simulink model "strain_gauge"  (R2019b)
settings: Solver=ode15s  StartTime=0.0  StopTime=100  RelTol=1e-3  AbsTol=1e-3  EnableMultiTasking=on
libraries: fl_lib x13, ee_lib x6, nesl_utility x3, simulink x1, dspsigops x1
Description:
  | Strain Gauge and Wheatstone Bridge
settings Model: ExtModeAutoUpdateStatusClock=off  Creator=The MathWorks, Inc.  LastModifiedBy=upattacini
settings SolverCC: AutoScaleAbsTol=off
settings DataIOCC: MaxDataPoints=10000  SaveOutput=off  SignalLogging=off  DSMLogging=off  SaveTime=off  ReturnWorkspaceOutputs=off  SignalLoggingName=logsout_ee_strain_gauge  Refine=5
settings OptimizationCC: ExpressionDepthLimit=2147483647  InitFltsAndDblsToZero=on  LifeSpan=inf
settings DebuggingCC: SaveWithParameterizedLinksMsg=none  UnderspecifiedInitializationDetection=Classic  MergeDetectMultiDrivingBlocksExec=none  SignalResolutionControl=TryResolveAllWithWarning  FcnCallInpInsideContextMsg=warning  StateNameClashWarn=warning  SFUnexpectedBacktrackingDiag=warning  SFNoUnconditionalDefaultTransitionDiag=warning  SFExecutionAtInitializationDiag=none  ArithmeticOperatorsInVariantConditions=warning
settings HardwareCC: ProdBitPerPointer=32  ProdBitPerSizeT=32  ProdBitPerPtrDiffT=32  ProdLargestAtomicFloat=None  ProdIntDivRoundTo=Undefined  ProdEndianess=Unspecified  ProdWordSize=32  ProdHWDeviceType=32-bit Generic
settings ModelReferenceCC: PropagateSignalLabelsOutOfModel=off
settings SFSimCC: SimUseLocalCustomCode=off  CustomCodeUndefinedFunction=UseInterfaceOnly
settings RTWCC: RTWUseLocalCustomCode=off
settings CodeAppCC: StateflowObjectComments=on
settings GRTTargetCC: TargetFcnLib=ansi_tfl_tmw.mat  TargetLangStandard=C89/C90 (ANSI)  GeneratePreprocessorConditionals=Disable all  CombineOutputUpdateFcns=off  GRTInterface=on
settings ConfigComp: CovMetricSettings=dw  CovHtmlReporting=on  CovSaveCumulativeToWorkspaceVar=on  CovSaveSingleToWorkspaceVar=on  CovExternalEMLEnable=off  CovSFcnEnable=off
settings SimscapeCC: SimscapeLogName=simlog_ee_strain_gauge  SimscapeLogDataHistory=10000

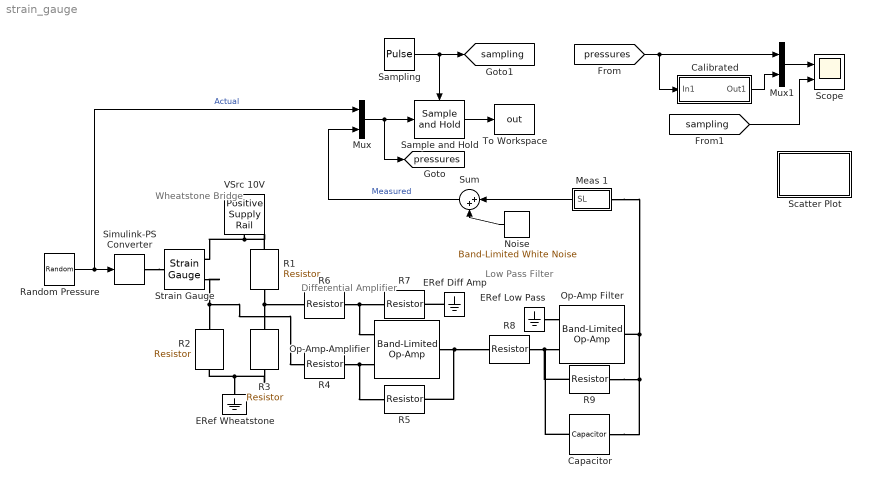
== system strain_gauge ==
  note: Low Pass Filter
  note: Differential Amplifier
  note: Wheatstone
      | Bridge
  Calibrated : Subsystem  mask{Switch=off, Gain=0.838, Bias=-8.5e-6}
      mask prompts: Switch "Enable Calibration"
      mask Callback Switch:
      | sw = get_param(gcb,'Switch');
      | if strcmp(sw,'on')
      |     set_param(gcb,'MaskEnableString','on,on,on');
      | else
      |     set_param(gcb,'MaskEnableString','on,off,off');
      | end
      mask DialogControl DescGroupVar Prompt: Calibration
      mask Display: disp('Calibration');
  Capacitor : ee_lib/Passive/Capacitor  cap_option=0  c=1e-6 F  Cvec=[ 1e-5 1e-6 ] F  Vvec=[ 0 10 ] V  CV_table_symmetry=1  f_vec=[1, 10] kHz  DFext_vec=[.8, 1.2]  C_tol=10  enable_C_tol=2  tol_distribution=1  nSigma=4  r=1e-6 Ohm  g=0 1/Ohm  averaging_period=0 s  enable_operating_limits=0  operating_limit_action=2  max_working_voltage_range=[ -25 25 ] V  power_rating=1 W  enable_faults=0  fault_action=1  Cscale_faulted=100  R_faulted=0.001 Ohm  G_faulted=0 1/Ohm  tau_fault=0.001 s  enable_temporal_fault=0  t_fault=1 s  enable_behavioral_fault=0  max_permissible_voltage_range=[ -100 100 ] V  t_fail_on_voltage=1 s  i_specify=off  i_priority=None  i=0 A  i_nominal_specify=off  i_nominal_unit=A  i_nominal_value=1  v_specify=off  v_priority=None  v=0 V  v_nominal_specify=off  v_nominal_unit=V  v_nominal_value=1  vc_specify=on  vc_priority=High  vc=0 V  vc_nominal_specify=off  vc_nominal_unit=V  vc_nominal_value=1
      settings: SourceProductName=Simscape Electrical
  ERef Diff Amp : fl_lib/Electrical/Electrical Elements/Electrical Reference
  ERef Low Pass : fl_lib/Electrical/Electrical Elements/Electrical Reference
  ERef Wheatstone : fl_lib/Electrical/Electrical Elements/Electrical Reference
  Meas 1 : Subsystem
  Mux : Mux  Inputs=2
  Mux1 : Mux  Inputs=2
  Noise : simulink/Sources/Band-Limited White Noise  Cov=2e-13  Ts=0.001  seed=[23341]
  Op-Amp Amplifier : ee_lib/Integrated Circuits/Band-Limited Op-Amp  A=1000  Rin=1e+06 Ohm  Rout=100 Ohm  Vmin=-15 V  Vmax=15 V  Vdotmax=1000 V/s  f=1e5 Hz  V0=0 V
      settings: SourceProductName=Simscape Electrical  SourceProductBaseCode=PS
  Op-Amp Filter : ee_lib/Integrated Circuits/Band-Limited Op-Amp  A=1000  Rin=1e+06 Ohm  Rout=100 Ohm  Vmin=-15 V  Vmax=15 V  Vdotmax=1000 V/s  f=1e5 Hz  V0=0 V
      settings: SourceProductName=Simscape Electrical  SourceProductBaseCode=PS
  R1 : fl_lib/Electrical/Electrical Elements/Resistor  R=100 Ohm  i_specify=off  i_priority=High  i=0 A  i_nominal_specify=off  i_nominal_unit=A  i_nominal_value=1  v_specify=off  v_priority=High  v=0 V  v_nominal_specify=off  v_nominal_unit=V  v_nominal_value=1
  R2 : fl_lib/Electrical/Electrical Elements/Resistor  R=100 Ohm  i_specify=off  i_priority=High  i=0 A  i_nominal_specify=off  i_nominal_unit=A  i_nominal_value=1  v_specify=off  v_priority=High  v=0 V  v_nominal_specify=off  v_nominal_unit=V  v_nominal_value=1
  R3 : fl_lib/Electrical/Electrical Elements/Resistor  R=100 Ohm  i_specify=off  i_priority=High  i=0 A  i_nominal_specify=off  i_nominal_unit=A  i_nominal_value=1  v_specify=off  v_priority=High  v=0 V  v_nominal_specify=off  v_nominal_unit=V  v_nominal_value=1
  R{4..7} (4 alike) : fl_lib/Electrical/Electrical Elements/Resistor  R=10 kOhm  i_specify=off  i_priority=High  i=0 A  i_nominal_specify=off  i_nominal_unit=A  i_nominal_value=1  v_specify=off  v_priority=High  v=0 V  v_nominal_specify=off  v_nominal_unit=V  v_nominal_value=1
  R8 : fl_lib/Electrical/Electrical Elements/Resistor  R=1 kOhm  i_specify=off  i_priority=High  i=0 A  i_nominal_specify=off  i_nominal_unit=A  i_nominal_value=1  v_specify=off  v_priority=High  v=0 V  v_nominal_specify=off  v_nominal_unit=V  v_nominal_value=1
  R9 : ee_lib/Passive/Resistor  R=100 kOhm  R_tol=20  enable_R_tol=2  tol_distribution=1  nSigma=4  enable_operating_limits=0  operating_limit_action=2  max_working_voltage=100 V  power_rating=1 W  enable_faults=0  fault_action=1  R_faulted=Inf Ohm  enable_temporal_fault=0  t_fault=1 s  enable_behavioral_fault=0  max_permissible_current=1 A  t_fail_on_current=1 s  noise_mode=0  sample_time=0.001 s  repeatability=1  auto_seed=3646982598  user_seed=0  Tdevice=25 degC  alpha=3.93e-3 1/K  Tmeas=25 degC  thermal_mass=100 J/K  power_derating_T1=70 degC  power_derating_T2=155 degC  operating_temperature_range_vec=[-50, 150] degC  temperature_specify=off  temperature_priority=High  temperature=298.15 K  temperature_nominal_specify=off  temperature_nominal_unit=K  temperature_nominal_value=1
      settings: SourceProductName=Simscape Electrical
  "Random Pressure " : UniformRandomNumber  Minimum=0  Maximum=0.001  SampleTime=1
  Sample and Hold : dspsigops/Sample and Hold  trig=Rising edge  initCond=0  latchinput=off
  Sampling : DiscretePulseGenerator  PulseType=Time based  Amplitude=1e-4  Period=1  PhaseDelay=0.9
  Scatter Plot : Subsystem
      settings: OpenFcn=|
      | if exist('out','var')
      |   figure('color','w');
      |   scatter(out(2:end,2),out(2:end,1));
      |   axis('equal');
      |   grid('on');
      |   title('Scatter Plot');
      |   xlabel('Measured');
      |   ylabel('Actual');
      | else
      |   warndlg('No data found in the workspace. Please run the simulation first.');
      | end
      mask Display: disp('Scatter Plot');
  Scope : Scope  NumInputPorts=2
  Simulink-PS Converter : nesl_utility/Simulink-PS Converter  PhysicalDomain=network_engine_domain  SubClassName=ps_input  LeftPortType=input  RightPortType=output  PseudoPeriodic=off  Frequencies=[]  NoiseDistribution=none  NoiseParameters=[]  Unit=1  AffineConversion=off  FilteringAndDerivatives=zero  SimscapeFilterOrder=1  InputFilterTimeConstant=.001  UdotUserProvided=0
  Strain Gauge : ee_lib/Sensors & Transducers/Strain Gauge  R=100 Ohm  K=2
      settings: SourceProductName=Simscape Electrical  SourceProductBaseCode=PS  InternalSimscapePortConfiguration="{\"Bottom\":[],\"Left\":[{\"id\":\"E\",\"label\":\"E\",\"type\":\"input\"}],\"Right\":[{\"id\":\"p\",\"label\":\"+\",\"type\":\"foundation.electrical.electrical\"},{\"id\":\"n\",\"label\":\"-\",\"type\":\"foundation.electrical.electrical\"}],\"Top\":[]}"
  Sum : Sum  Inputs=|++
  To Workspace : ToWorkspace  VariableName=out  SampleTime=1
      settings: Save2DSignal=2-D array (concatenate along first dimension)
  VSrc 10V : ee_lib/Sources/Positive Supply Rail  v0=10 V
      settings: SourceProductName=Simscape Electrical  SourceProductBaseCode=PS  InternalSimscapePortConfiguration="{\"Bottom\":[],\"Left\":[],\"Right\":[{\"id\":\"p\",\"label\":\"\",\"type\":\"foundation.electrical.electrical\"}],\"Top\":[]}"
  tag scope: pressures=global, sampling=global
  wires:
  "Random Pressure "/1 -> Simulink-PS Converter/1, Mux/1  "Actual"
  Mux/1 -> [pressures], Sample and Hold/1
  Sample and Hold/1 -> To Workspace/1
  Meas 1/1(SL) -> Sum/1
  Sum/1 -> Mux/2  "Measured"
  Noise/1 -> Sum/2
  [sampling] -> Scope/2
  [pressures] -> Calibrated/1(In1), Mux1/1
  Mux1/1 -> Scope/1
  Sampling/1 -> [sampling], Sample and Hold/Trigger
  Calibrated/1(Out1) -> Mux1/2
  connections:
  R1/LConn1 -- Strain Gauge/RConn1 -- VSrc 10V/RConn1
  Strain Gauge/RConn2 -- R4/LConn1 -- R2/LConn1
  R1/RConn1 -- R6/LConn1 -- R3/LConn1
  R3/RConn1 -- R2/RConn1 -- ERef Wheatstone/LConn1
  R4/RConn1 -- R5/LConn1 -- Op-Amp Amplifier/LConn2
  Op-Amp Amplifier/RConn1 -- R5/RConn1 -- R8/LConn1
  R6/RConn1 -- R7/LConn1 -- Op-Amp Amplifier/LConn1
  ERef Diff Amp/LConn1 -- R7/RConn1
  R9/RConn1 -- Meas 1/LConn1 -- Op-Amp Filter/RConn1 -- Capacitor/RConn1
  Simulink-PS Converter/RConn1 -- Strain Gauge/LConn1
  R8/RConn1 -- Capacitor/LConn1 -- R9/LConn1 -- Op-Amp Filter/LConn2
  ERef Low Pass/LConn1 -- Op-Amp Filter/LConn1

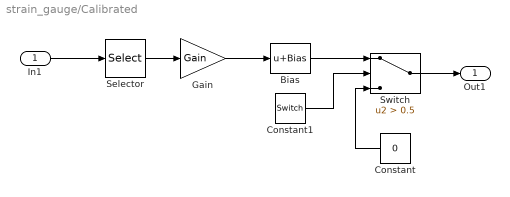
== system strain_gauge/Calibrated ==
  In1 : Inport
  Bias : Bias  Bias=Bias
  Constant : Constant  Value=0
  Constant1 : Constant  Value=Switch
  Gain : Gain  Gain=Gain
  Selector : Selector  InputPortWidth=2  IndexOptions=Index vector (dialog)  Indices=2  OutputSizes=1
  Switch : Switch  Criteria=u2 > Threshold  Threshold=0.5
  Out1 : Outport
  wires:
  In1/1 -> Selector/1
  Gain/1 -> Bias/1
  Selector/1 -> Gain/1
  Bias/1 -> Switch/1
  Constant/1 -> Switch/3
  Constant1/1 -> Switch/2
  Switch/1 -> Out1/1

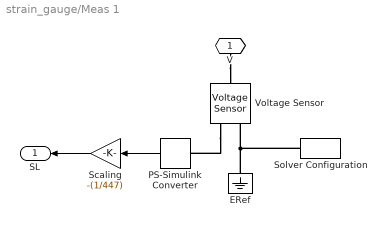
== system strain_gauge/Meas 1 ==
  ERef : fl_lib/Electrical/Electrical Elements/Electrical Reference
  PS-Simulink Converter : nesl_utility/PS-Simulink Converter  PhysicalDomain=network_engine_domain  SubClassName=ps_output  LeftPortType=input  RightPortType=output  PseudoPeriodic=off  Frequencies=[]  Unit=V  AffineConversion=off
  Scaling : Gain  Gain=-(1/447)
  Solver Configuration : nesl_utility/Solver Configuration  PhysicalDomain=network_engine_domain  SubClassName=solver  LeftPortType=input  RightPortType=generic  Tones=[]  Harmonics=[]  SimulateNoise=off  Profile=off  UseLocalSampling=off  EnableSwitchedLinearOptims=on  FrequencyDomain=off  UseCCode=off  RelTol=0.001  AbsTol=1e-06  MinStep=1e-09  ToWorkspace=off  RevertToSquareIcSolve=off  NumHomotopyIterations=100  PhasorMode=off  PhasorModeNumHarmonics=1  DoDC=off  ResidualTolerance=1e-9  UseLocalSolver=off  LocalSolverChoice=NE_BACKWARD_EULER_ADVANCER  LocalSolverSampleTime=.001  DoFixedCost=off  MaxNonlinIter=3  MaxModeIter=2  LinearAlgebra=auto  EquationFormulation=NE_TIME_EF  DelaysMemoryBudget=1024  AutomaticFiltering=on  FilteringTimeConstant=0.001  PartitionStorageMethod=AS_NEEDED  PartitionMemoryBudget=1024  PartitionMethod=FAST
  Voltage Sensor : fl_lib/Electrical/Electrical Sensors/Voltage Sensor
  V : PMIOPort  Side=Left
  SL : Outport  VectorParamsAs1DForOutWhenUnconnected=off
  wires:
  PS-Simulink Converter/1 -> Scaling/1
  Scaling/1 -> SL/1
  connections:
  V/RConn1 -- Voltage Sensor/LConn1
  ERef/LConn1 -- Solver Configuration/RConn1 -- Voltage Sensor/RConn2
  Voltage Sensor/RConn1 -- PS-Simulink Converter/LConn1

== system strain_gauge/Scatter Plot ==
